simulink subsystem "sscfluids_ev_battery_cooling_variant"  (R2024a)
settings: Solver=VariableStepAuto  StartTime=0.0  StopTime=10.0  RelTol=1e-3
undefined symbols (not defined in the file): BattTempInit, pipe, pump, radiator, T_env, T_set, tank, valve
libraries: fl_lib x101, nesl_utility_internal x25, SimscapeFluids_lib x7, slpidlib x1, simulink_extras x1
(part 3 of 3)

== system sscfluids_ev_battery_cooling_variant/Cold Plate/One-Pass/Cooling Plate (Pack 1) ==
  Battery to plate conduction : fl_lib/Thermal/Thermal Elements/Conductive Heat Transfer  thermal_type=foundation.enum.ConstantVariableTabulated.Constant  wall_geometry=foundation.enum.ConductionWallGeometry.Planar  area=0.5*2 m^2  thickness=1 mm  d_in=0.05 m  d_out=0.1 m  L=1 m  th_cond_min=10 W/(K*m)  th_cond=205 W/(m*K)  th_cond_TLU=[413, 401, 392, 383, 371, 357, 342] W/(K*m)  temp_TLU=[200, 273, 400, 600, 800, 1000, 1200] K  T_specify=off  T_priority=None  T=0 K  T_nominal_specify=off  T_nominal_value=1  T_nominal_unit=K  Q_specify=off  Q_priority=None  Q=0 W  Q_nominal_specify=off  Q_nominal_value=1  Q_nominal_unit=W
  First Order Hold1 : FirstOrderHold  ErrorTolerance=inf  AllowContinuousInput=on
  Heat Flow Rate Sensor : fl_lib/Thermal/Thermal Sensors/Heat Flow Rate Sensor
  PS-Simulink Converter2 : nesl_utility_internal/PS-Simulink Converter  PhysicalDomain=network_engine_domain  SubClassName=ps_output  LeftPortType=input  RightPortType=output  PseudoPeriodic=off  Frequencies=[]  VectorFormat=inherit  Unit=inherit  AffineConversion=off
  "Plate mass " : fl_lib/Thermal/Thermal Elements/Thermal Mass  mass_type=foundation.enum.constant_variable.constant  mass=10*2 kg  sp_heat=910 J/kg/K  mass_min=1e-6 kg  num_ports=foundation.enum.numPorts2.one  m_specify=off  m_priority=High  m=1 kg  m_nominal_specify=off  m_nominal_value=1  m_nominal_unit=kg  T_specify=on  T_priority=High  T=BattTempInit degC  T_nominal_specify=off  T_nominal_value=1  T_nominal_unit=K  Q_specify=off  Q_priority=None  Q=0 W  Q_nominal_specify=off  Q_nominal_value=1  Q_nominal_unit=W
  Reshape : Reshape
  H1 : PMIOPort  Side=Left
  T1 : PMIOPort  Port=2  Side=Right
  tag scope: Pcp1=global
  wires:
  First Order Hold1/1 -> [Pcp1]  "Pcp1FOH"
  Reshape/1 -> First Order Hold1/1
  PS-Simulink Converter2/1 -> Reshape/1  "Pcp1"
  connections:
  Heat Flow Rate Sensor/RConn2 -- Battery to plate conduction/LConn1
  Heat Flow Rate Sensor/LConn1 -- T1/RConn1
  PS-Simulink Converter2/LConn1 -- Heat Flow Rate Sensor/RConn1
  "Plate mass "/LConn1 -- H1/RConn1 -- Battery to plate conduction/RConn1

== system sscfluids_ev_battery_cooling_variant/Cold Plate/One-Pass/Cooling Plate (Pack 2) ==
  Battery to plate conduction : fl_lib/Thermal/Thermal Elements/Conductive Heat Transfer  thermal_type=foundation.enum.ConstantVariableTabulated.Constant  wall_geometry=foundation.enum.ConductionWallGeometry.Planar  area=0.5*2 m^2  thickness=1 mm  d_in=0.05 m  d_out=0.1 m  L=1 m  th_cond_min=10 W/(K*m)  th_cond=205 W/(m*K)  th_cond_TLU=[413, 401, 392, 383, 371, 357, 342] W/(K*m)  temp_TLU=[200, 273, 400, 600, 800, 1000, 1200] K  T_specify=off  T_priority=None  T=0 K  T_nominal_specify=off  T_nominal_value=1  T_nominal_unit=K  Q_specify=off  Q_priority=None  Q=0 W  Q_nominal_specify=off  Q_nominal_value=1  Q_nominal_unit=W
  First Order Hold1 : FirstOrderHold  ErrorTolerance=inf  AllowContinuousInput=on
  Heat Flow Rate Sensor : fl_lib/Thermal/Thermal Sensors/Heat Flow Rate Sensor
  PS-Simulink Converter2 : nesl_utility_internal/PS-Simulink Converter  PhysicalDomain=network_engine_domain  SubClassName=ps_output  LeftPortType=input  RightPortType=output  PseudoPeriodic=off  Frequencies=[]  VectorFormat=inherit  Unit=inherit  AffineConversion=off
  "Plate mass " : fl_lib/Thermal/Thermal Elements/Thermal Mass  mass_type=foundation.enum.constant_variable.constant  mass=10*2 kg  sp_heat=910 J/kg/K  mass_min=1e-6 kg  num_ports=foundation.enum.numPorts2.one  m_specify=off  m_priority=High  m=1 kg  m_nominal_specify=off  m_nominal_value=1  m_nominal_unit=kg  T_specify=on  T_priority=High  T=BattTempInit degC  T_nominal_specify=off  T_nominal_value=1  T_nominal_unit=K  Q_specify=off  Q_priority=None  Q=0 W  Q_nominal_specify=off  Q_nominal_value=1  Q_nominal_unit=W
  Reshape : Reshape
  H1 : PMIOPort  Side=Left
  T2 : PMIOPort  Port=2  Side=Right
  tag scope: Pcp2=global
  wires:
  First Order Hold1/1 -> [Pcp2]
  Reshape/1 -> First Order Hold1/1
  PS-Simulink Converter2/1 -> Reshape/1
  connections:
  Heat Flow Rate Sensor/RConn2 -- Battery to plate conduction/LConn1
  Heat Flow Rate Sensor/LConn1 -- T2/RConn1
  PS-Simulink Converter2/LConn1 -- Heat Flow Rate Sensor/RConn1
  "Plate mass "/LConn1 -- H1/RConn1 -- Battery to plate conduction/RConn1

== system sscfluids_ev_battery_cooling_variant/Cold Plate/One-Pass/Cooling Plate (Pack 3) ==
  Battery to plate conduction : fl_lib/Thermal/Thermal Elements/Conductive Heat Transfer  thermal_type=foundation.enum.ConstantVariableTabulated.Constant  wall_geometry=foundation.enum.ConductionWallGeometry.Planar  area=0.5*2 m^2  thickness=1 mm  d_in=0.05 m  d_out=0.1 m  L=1 m  th_cond_min=10 W/(K*m)  th_cond=205 W/(m*K)  th_cond_TLU=[413, 401, 392, 383, 371, 357, 342] W/(K*m)  temp_TLU=[200, 273, 400, 600, 800, 1000, 1200] K  T_specify=off  T_priority=None  T=0 K  T_nominal_specify=off  T_nominal_value=1  T_nominal_unit=K  Q_specify=off  Q_priority=None  Q=0 W  Q_nominal_specify=off  Q_nominal_value=1  Q_nominal_unit=W
  First Order Hold1 : FirstOrderHold  ErrorTolerance=inf  AllowContinuousInput=on
  Heat Flow Rate Sensor : fl_lib/Thermal/Thermal Sensors/Heat Flow Rate Sensor
  PS-Simulink Converter2 : nesl_utility_internal/PS-Simulink Converter  PhysicalDomain=network_engine_domain  SubClassName=ps_output  LeftPortType=input  RightPortType=output  PseudoPeriodic=off  Frequencies=[]  VectorFormat=inherit  Unit=inherit  AffineConversion=off
  "Plate mass " : fl_lib/Thermal/Thermal Elements/Thermal Mass  mass_type=foundation.enum.constant_variable.constant  mass=10*2 kg  sp_heat=910 J/kg/K  mass_min=1e-6 kg  num_ports=foundation.enum.numPorts2.one  m_specify=off  m_priority=High  m=1 kg  m_nominal_specify=off  m_nominal_value=1  m_nominal_unit=kg  T_specify=on  T_priority=High  T=BattTempInit degC  T_nominal_specify=off  T_nominal_value=1  T_nominal_unit=K  Q_specify=off  Q_priority=None  Q=0 W  Q_nominal_specify=off  Q_nominal_value=1  Q_nominal_unit=W
  Reshape : Reshape
  H1 : PMIOPort  Side=Left
  T3 : PMIOPort  Port=2  Side=Right
  tag scope: Pcp3=global
  wires:
  First Order Hold1/1 -> [Pcp3]
  Reshape/1 -> First Order Hold1/1
  PS-Simulink Converter2/1 -> Reshape/1  "Pcp3"
  connections:
  T3/RConn1 -- Heat Flow Rate Sensor/LConn1
  PS-Simulink Converter2/LConn1 -- Heat Flow Rate Sensor/RConn1
  Heat Flow Rate Sensor/RConn2 -- Battery to plate conduction/LConn1
  Battery to plate conduction/RConn1 -- H1/RConn1 -- "Plate mass "/LConn1

== system sscfluids_ev_battery_cooling_variant/Cold Plate/One-Pass/Cooling Plate (Pack 4) ==
  Battery to plate conduction : fl_lib/Thermal/Thermal Elements/Conductive Heat Transfer  thermal_type=foundation.enum.ConstantVariableTabulated.Constant  wall_geometry=foundation.enum.ConductionWallGeometry.Planar  area=0.5*2 m^2  thickness=1 mm  d_in=0.05 m  d_out=0.1 m  L=1 m  th_cond_min=10 W/(K*m)  th_cond=205 W/(m*K)  th_cond_TLU=[413, 401, 392, 383, 371, 357, 342] W/(K*m)  temp_TLU=[200, 273, 400, 600, 800, 1000, 1200] K  T_specify=off  T_priority=None  T=0 K  T_nominal_specify=off  T_nominal_value=1  T_nominal_unit=K  Q_specify=off  Q_priority=None  Q=0 W  Q_nominal_specify=off  Q_nominal_value=1  Q_nominal_unit=W
  First Order Hold1 : FirstOrderHold  ErrorTolerance=inf  AllowContinuousInput=on
  Heat Flow Rate Sensor : fl_lib/Thermal/Thermal Sensors/Heat Flow Rate Sensor
  PS-Simulink Converter2 : nesl_utility_internal/PS-Simulink Converter  PhysicalDomain=network_engine_domain  SubClassName=ps_output  LeftPortType=input  RightPortType=output  PseudoPeriodic=off  Frequencies=[]  VectorFormat=inherit  Unit=inherit  AffineConversion=off
  "Plate mass " : fl_lib/Thermal/Thermal Elements/Thermal Mass  mass_type=foundation.enum.constant_variable.constant  mass=10*2 kg  sp_heat=910 J/kg/K  mass_min=1e-6 kg  num_ports=foundation.enum.numPorts2.one  m_specify=off  m_priority=High  m=1 kg  m_nominal_specify=off  m_nominal_value=1  m_nominal_unit=kg  T_specify=on  T_priority=High  T=BattTempInit degC  T_nominal_specify=off  T_nominal_value=1  T_nominal_unit=K  Q_specify=off  Q_priority=None  Q=0 W  Q_nominal_specify=off  Q_nominal_value=1  Q_nominal_unit=W
  Reshape : Reshape
  H1 : PMIOPort  Side=Left
  T4 : PMIOPort  Port=2  Side=Right
  tag scope: Pcp4=global
  wires:
  First Order Hold1/1 -> [Pcp4]
  Reshape/1 -> First Order Hold1/1
  PS-Simulink Converter2/1 -> Reshape/1  "Pcp4"
  connections:
  Heat Flow Rate Sensor/RConn1 -- PS-Simulink Converter2/LConn1
  Heat Flow Rate Sensor/RConn2 -- Battery to plate conduction/LConn1
  T4/RConn1 -- Heat Flow Rate Sensor/LConn1
  "Plate mass "/LConn1 -- H1/RConn1 -- Battery to plate conduction/RConn1

== system sscfluids_ev_battery_cooling_variant/Cold Plate/One-Pass/Power Sensor1 ==
  First Order Hold1 : FirstOrderHold  ErrorTolerance=inf  AllowContinuousInput=on
  Mass & Energy Flow Rate Sensor (TL) : fl_lib/Thermal Liquid/Sensors/Flow Rate Sensor (TL)  mass_flow_measure=true  volumetric_flow_measure=false  energy_flow_measure=true
      settings: InternalSimscapePortConfiguration="{\"Bottom\":[{\"id\":\"PHI\",\"label\":\"φ\",\"type\":\"output\"}],\"Left\":[{\"id\":\"A\",\"label\":\"A\",\"type\":\"foundation.thermal_liquid.thermal_liquid\"}],\"Right\":[{\"id\":\"B\",\"label\":\"B\",\"type\":\"foundation.thermal_liquid.thermal_liquid\"},{\"id\":\"M\",\"label\":\"M\",\"type\":\"output\"}],\"Top\":[]}"
  PS-Simulink Converter2 : nesl_utility_internal/PS-Simulink Converter  PhysicalDomain=network_engine_domain  SubClassName=ps_output  LeftPortType=input  RightPortType=output  PseudoPeriodic=off  Frequencies=[]  VectorFormat=inherit  Unit=inherit  AffineConversion=off
  Reshape : Reshape
  B : PMIOPort  Side=Left
  A : PMIOPort  Port=2  Side=Right
  tag scope: Ppipe1=global
  wires:
  First Order Hold1/1 -> [Ppipe1]
  Reshape/1 -> First Order Hold1/1
  PS-Simulink Converter2/1 -> Reshape/1  "Ppipe1"
  connections:
  Mass & Energy Flow Rate Sensor (TL)/LConn1 -- A/RConn1
  Mass & Energy Flow Rate Sensor (TL)/RConn3 -- PS-Simulink Converter2/LConn1
  Mass & Energy Flow Rate Sensor (TL)/RConn1 -- B/RConn1

== system sscfluids_ev_battery_cooling_variant/Cold Plate/One-Pass/Power Sensor2 ==
  First Order Hold1 : FirstOrderHold  ErrorTolerance=inf  AllowContinuousInput=on
  Mass & Energy Flow Rate Sensor (TL) : fl_lib/Thermal Liquid/Sensors/Flow Rate Sensor (TL)  mass_flow_measure=true  volumetric_flow_measure=false  energy_flow_measure=true
      settings: InternalSimscapePortConfiguration="{\"Bottom\":[{\"id\":\"PHI\",\"label\":\"φ\",\"type\":\"output\"}],\"Left\":[{\"id\":\"A\",\"label\":\"A\",\"type\":\"foundation.thermal_liquid.thermal_liquid\"}],\"Right\":[{\"id\":\"B\",\"label\":\"B\",\"type\":\"foundation.thermal_liquid.thermal_liquid\"},{\"id\":\"M\",\"label\":\"M\",\"type\":\"output\"}],\"Top\":[]}"
  PS-Simulink Converter2 : nesl_utility_internal/PS-Simulink Converter  PhysicalDomain=network_engine_domain  SubClassName=ps_output  LeftPortType=input  RightPortType=output  PseudoPeriodic=off  Frequencies=[]  VectorFormat=inherit  Unit=inherit  AffineConversion=off
  Reshape : Reshape
  A : PMIOPort  Side=Left
  B : PMIOPort  Port=2  Side=Right
  tag scope: Ppipe2=global
  wires:
  First Order Hold1/1 -> [Ppipe2]
  Reshape/1 -> First Order Hold1/1
  PS-Simulink Converter2/1 -> Reshape/1  "Ppipe2"
  connections:
  Mass & Energy Flow Rate Sensor (TL)/RConn1 -- B/RConn1
  Mass & Energy Flow Rate Sensor (TL)/RConn3 -- PS-Simulink Converter2/LConn1
  Mass & Energy Flow Rate Sensor (TL)/LConn1 -- A/RConn1

== system sscfluids_ev_battery_cooling_variant/Cold Plate/One-Pass/Power Sensor3 ==
  First Order Hold1 : FirstOrderHold  ErrorTolerance=inf  AllowContinuousInput=on
  Mass & Energy Flow Rate Sensor (TL) : fl_lib/Thermal Liquid/Sensors/Flow Rate Sensor (TL)  mass_flow_measure=true  volumetric_flow_measure=false  energy_flow_measure=true
      settings: InternalSimscapePortConfiguration="{\"Bottom\":[{\"id\":\"PHI\",\"label\":\"φ\",\"type\":\"output\"}],\"Left\":[{\"id\":\"A\",\"label\":\"A\",\"type\":\"foundation.thermal_liquid.thermal_liquid\"}],\"Right\":[{\"id\":\"B\",\"label\":\"B\",\"type\":\"foundation.thermal_liquid.thermal_liquid\"},{\"id\":\"M\",\"label\":\"M\",\"type\":\"output\"}],\"Top\":[]}"
  PS-Simulink Converter2 : nesl_utility_internal/PS-Simulink Converter  PhysicalDomain=network_engine_domain  SubClassName=ps_output  LeftPortType=input  RightPortType=output  PseudoPeriodic=off  Frequencies=[]  VectorFormat=inherit  Unit=inherit  AffineConversion=off
  Reshape : Reshape
  A : PMIOPort  Side=Left
  B : PMIOPort  Port=2  Side=Right
  tag scope: Pcvc1=global
  wires:
  First Order Hold1/1 -> [Pcvc1]
  Reshape/1 -> First Order Hold1/1
  PS-Simulink Converter2/1 -> Reshape/1  "Pcvc1"
  connections:
  Mass & Energy Flow Rate Sensor (TL)/LConn1 -- A/RConn1
  Mass & Energy Flow Rate Sensor (TL)/RConn3 -- PS-Simulink Converter2/LConn1
  Mass & Energy Flow Rate Sensor (TL)/RConn1 -- B/RConn1

== system sscfluids_ev_battery_cooling_variant/Cold Plate/One-Pass/Power Sensor4 ==
  First Order Hold2 : FirstOrderHold  ErrorTolerance=inf  AllowContinuousInput=on
  Mass & Energy Flow Rate Sensor (TL) : fl_lib/Thermal Liquid/Sensors/Flow Rate Sensor (TL)  mass_flow_measure=true  volumetric_flow_measure=false  energy_flow_measure=true
      settings: InternalSimscapePortConfiguration="{\"Bottom\":[{\"id\":\"PHI\",\"label\":\"φ\",\"type\":\"output\"}],\"Left\":[{\"id\":\"A\",\"label\":\"A\",\"type\":\"foundation.thermal_liquid.thermal_liquid\"}],\"Right\":[{\"id\":\"B\",\"label\":\"B\",\"type\":\"foundation.thermal_liquid.thermal_liquid\"},{\"id\":\"M\",\"label\":\"M\",\"type\":\"output\"}],\"Top\":[]}"
  PS-Simulink Converter2 : nesl_utility_internal/PS-Simulink Converter  PhysicalDomain=network_engine_domain  SubClassName=ps_output  LeftPortType=input  RightPortType=output  PseudoPeriodic=off  Frequencies=[]  VectorFormat=inherit  Unit=inherit  AffineConversion=off
  Reshape : Reshape
  A : PMIOPort  Side=Left
  B : PMIOPort  Port=2  Side=Right
  tag scope: Ppipe4=global
  wires:
  First Order Hold2/1 -> [Ppipe4]
  Reshape/1 -> First Order Hold2/1
  PS-Simulink Converter2/1 -> Reshape/1  "Ppipe4"
  connections:
  Mass & Energy Flow Rate Sensor (TL)/RConn1 -- B/RConn1
  Mass & Energy Flow Rate Sensor (TL)/RConn3 -- PS-Simulink Converter2/LConn1
  Mass & Energy Flow Rate Sensor (TL)/LConn1 -- A/RConn1

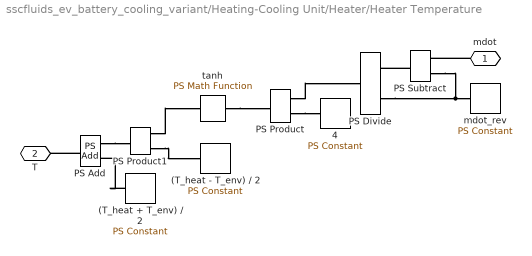
== system sscfluids_ev_battery_cooling_variant/Heating-Cooling Unit/Heater/Heater Temperature ==
  (T_heat + T_env) / 2 : fl_lib/Physical Signals/Sources/PS Constant  constant=(T_heat +T_env + 273.15)/2 K
  (T_heat - T_env) / 2 : fl_lib/Physical Signals/Sources/PS Constant  constant=(T_heat - T_env - 273.15)/2 K
  4 : fl_lib/Physical Signals/Sources/PS Constant  constant=4
  PS Add : fl_lib/Physical Signals/Functions/PS Add
  PS Divide : fl_lib/Physical Signals/Functions/PS Divide
  PS Product : fl_lib/Physical Signals/Functions/PS Product
  PS Product1 : fl_lib/Physical Signals/Functions/PS Product
  PS Subtract : fl_lib/Physical Signals/Functions/PS Subtract
  mdot_rev : fl_lib/Physical Signals/Sources/PS Constant  constant=mdot_rev kg/s
  tanh : fl_lib/Physical Signals/Functions/PS Math Function  fcn_choice=foundation.enum.math_function.tanh  v=1
  mdot : PMIOPort  Side=Left
  T : PMIOPort  Port=2  Side=Right
  connections:
  PS Add/RConn1 -- T/RConn1
  tanh/LConn1 -- PS Product/RConn1
  PS Divide/LConn2 -- PS Subtract/LConn2 -- mdot_rev/RConn1
  PS Product/LConn2 -- 4/RConn1
  PS Add/LConn1 -- PS Product1/RConn1
  PS Subtract/RConn1 -- PS Divide/LConn1
  PS Product1/LConn2 -- (T_heat - T_env) / 2/RConn1
  PS Product1/LConn1 -- tanh/RConn1
  PS Product/LConn1 -- PS Divide/RConn1
  (T_heat + T_env) / 2/RConn1 -- PS Add/LConn2
  mdot/RConn1 -- PS Subtract/LConn1

== system sscfluids_ev_battery_cooling_variant/Heating-Cooling Unit/Heater/Power Sensor ==
  First Order Hold1 : FirstOrderHold  ErrorTolerance=inf  AllowContinuousInput=on
  Heat Flow Rate Sensor : fl_lib/Thermal/Thermal Sensors/Heat Flow Rate Sensor
  PS-Simulink Converter2 : nesl_utility_internal/PS-Simulink Converter  PhysicalDomain=network_engine_domain  SubClassName=ps_output  LeftPortType=input  RightPortType=output  PseudoPeriodic=off  Frequencies=[]  VectorFormat=inherit  Unit=inherit  AffineConversion=off
  Reshape : Reshape
  A : PMIOPort  Side=Left
  B : PMIOPort  Port=2  Side=Right
  tag scope: PhHeater=global
  wires:
  First Order Hold1/1 -> [PhHeater]
  Reshape/1 -> First Order Hold1/1
  PS-Simulink Converter2/1 -> Reshape/1  "PhHeater"
  connections:
  Heat Flow Rate Sensor/LConn1 -- A/RConn1
  Heat Flow Rate Sensor/RConn2 -- B/RConn1
  PS-Simulink Converter2/LConn1 -- Heat Flow Rate Sensor/RConn1

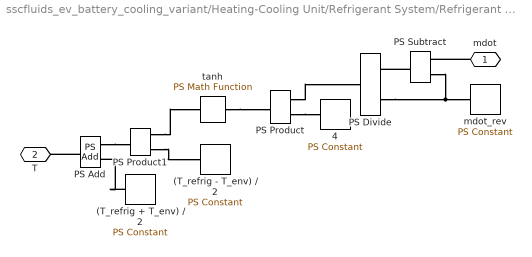
== system sscfluids_ev_battery_cooling_variant/Heating-Cooling Unit/Refrigerant System/Refrigerant Temperature ==
  (T_refrig + T_env) / 2 : fl_lib/Physical Signals/Sources/PS Constant  constant=(T_refrig+T_env+273.15)/2 K
  (T_refrig - T_env) / 2 : fl_lib/Physical Signals/Sources/PS Constant  constant=(T_refrig-T_env-273.15)/2 K
  4 : fl_lib/Physical Signals/Sources/PS Constant  constant=4
  PS Add : fl_lib/Physical Signals/Functions/PS Add
  PS Divide : fl_lib/Physical Signals/Functions/PS Divide
  PS Product : fl_lib/Physical Signals/Functions/PS Product
  PS Product1 : fl_lib/Physical Signals/Functions/PS Product
  PS Subtract : fl_lib/Physical Signals/Functions/PS Subtract
  mdot_rev : fl_lib/Physical Signals/Sources/PS Constant  constant=mdot_rev kg/s
  tanh : fl_lib/Physical Signals/Functions/PS Math Function  fcn_choice=foundation.enum.math_function.tanh  v=1
  mdot : PMIOPort  Side=Left
  T : PMIOPort  Port=2  Side=Right
  connections:
  tanh/LConn1 -- PS Product/RConn1
  PS Product/LConn1 -- PS Divide/RConn1
  (T_refrig + T_env) / 2/RConn1 -- PS Add/LConn2
  PS Divide/LConn2 -- PS Subtract/LConn2 -- mdot_rev/RConn1
  PS Add/RConn1 -- T/RConn1
  PS Add/LConn1 -- PS Product1/RConn1
  PS Product1/LConn1 -- tanh/RConn1
  PS Product/LConn2 -- 4/RConn1
  PS Subtract/RConn1 -- PS Divide/LConn1
  PS Product1/LConn2 -- (T_refrig - T_env) / 2/RConn1
  mdot/RConn1 -- PS Subtract/LConn1
